simulink model "Prob4"  (R2020b)
settings: Solver=VariableStepAuto  StartTime=0.0  StopTime=10.0  RelTol=1e-3
model workspace (MAT data in the model file):
  a1 = Simulink.Parameter
  a1.Value = 0.5
  a1.DataType = 'auto'
  a1.Dimensions = [1 1]
  a2 = Simulink.Parameter
  a2.Value = -0.25
  a2.DataType = 'auto'
  a2.Dimensions = [1 1]
  b0 = Simulink.Parameter
  b0.Value = 1
  b0.DataType = 'auto'
  b0.Dimensions = [1 1]
  b1 = Simulink.Parameter
  b1.Value = 0.4
  b1.DataType = 'auto'
  b1.Dimensions = [1 1]
settings Model: OrderedModelArguments=off  Creator=shoun  LastModifiedBy=shoun

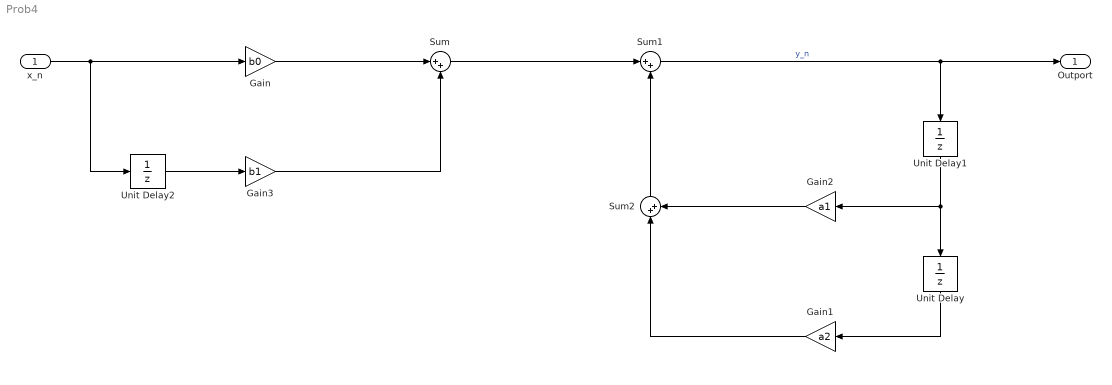
== system Prob4 ==
  x_n : Inport
  Gain : Gain  Gain=b0
  Gain1 : Gain  Gain=a2
  Gain2 : Gain  Gain=a1
  Gain3 : Gain  Gain=b1
  Sum : Sum  Inputs=|++
  Sum1 : Sum  Inputs=|++
  Sum2 : Sum  Inputs=|++
  Unit Delay : UnitDelay  SampleTime=-1  HasFrameUpgradeWarning=on
  Unit Delay1 : UnitDelay  SampleTime=-1  HasFrameUpgradeWarning=on
  Unit Delay2 : UnitDelay  SampleTime=-1  HasFrameUpgradeWarning=on
  Outport : Outport
  wires:
  x_n/1 -> Unit Delay2/1, Gain/1
  Gain/1 -> Sum/1
  Unit Delay2/1 -> Gain3/1
  Gain3/1 -> Sum/2
  Unit Delay1/1 -> Gain2/1, Unit Delay/1
  Unit Delay/1 -> Gain1/1
  Gain1/1 -> Sum2/1
  Gain2/1 -> Sum2/2
  Sum2/1 -> Sum1/2
  Sum/1 -> Sum1/1
  Sum1/1 -> Unit Delay1/1, Outport/1  "y_n"
